simulink model "TrajektorieAufbau"  (Simulink 4.00)
settings: Solver=ode4  StartTime=0.0  StopTime=1180  FixedStep=0.0100  RelTol=1e-3
undefined symbols (not defined in the file or in its folder): nedc

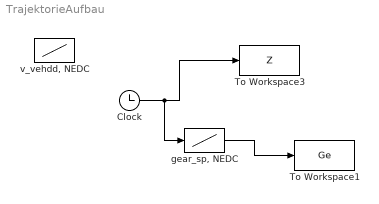
== system TrajektorieAufbau ==
  Clock : Clock
      settings: DisplayTime=off  Decimation=10
  To Workspace1 : ToWorkspace  VariableName=Ge  SampleTime=-1  SaveFormat=Array
  To Workspace3 : ToWorkspace  VariableName=Z  SampleTime=-1  SaveFormat=Array
  "gear_sp, NEDC" : Lookup  InputValues=nedc.gearshift_points(:,1)  OutputValues=nedc.gearshift_points(:,2)
  "v_vehdd, NEDC" : Lookup  InputValues=nedc.speed(:,1)  OutputValues=nedc.speed(:,2)
  wires:
  Clock/1 -> To Workspace3/1, "gear_sp, NEDC"/1
  "gear_sp, NEDC"/1 -> To Workspace1/1
